simulink model "sensorExpoler"  (R2026a)
settings: Solver=FixedStepDiscrete  StopTime=inf  FixedStep=0.001
undefined symbols (not defined in the file): Blocking, Non
libraries: amg_usbconverter_n_connect_lib x2
settings Model: Creator=pboon  LastModifiedBy=Next

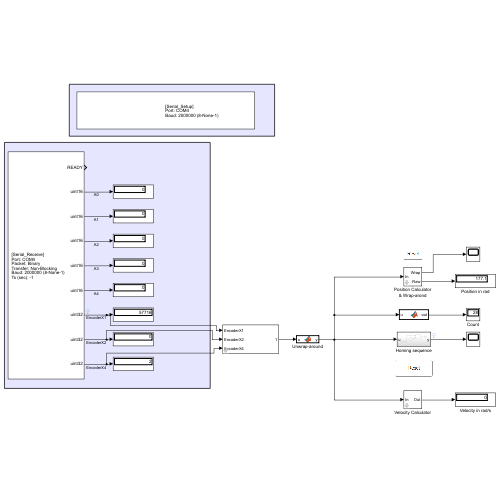
[thumbnail: Simulink's stored preview of the top-level diagram]
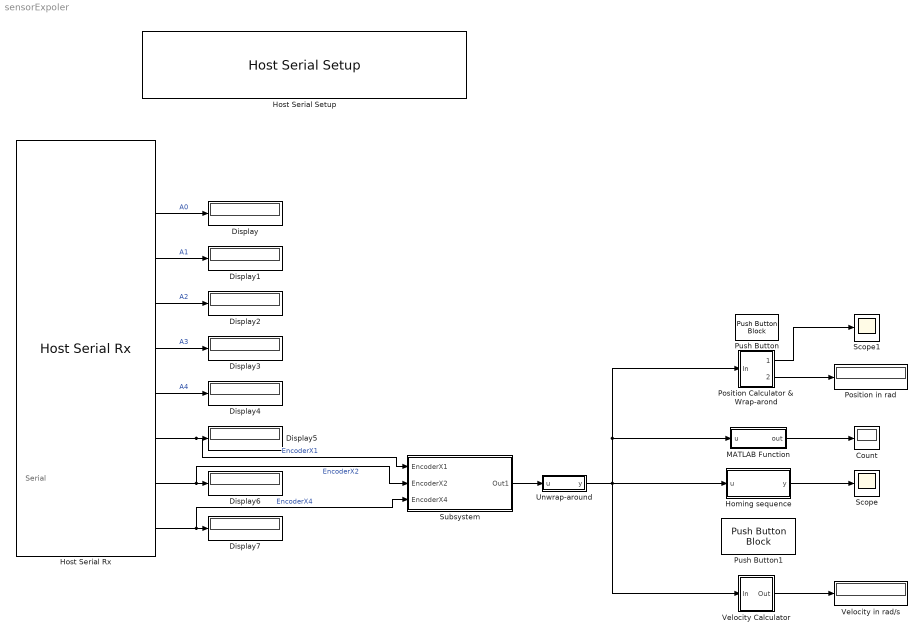
== system sensorExpoler ==
  note: Serial
  Count : Display
  Display{,1..7} (8 alike) : Display
      Display5 settings: Format=decimal (Stored Integer)
      Display6 settings: Format=decimal (Stored Integer)
      Display7 settings: Format=decimal (Stored Integer)
  Homing sequence : Subsystem
  Host Serial Rx : amg_usbconverter_n_connect_lib/Host Serial Rx  conf=rx  port=COM4  baudrate=2000000  databits=8  parity=None  stopbit=1  flowcontrol=None  transfer=Non-Blocking  timeout=5  packetmode=Binary  enableinitialvalues=off  initialvalues=[]  binheader='25'  binterminator='4E 4E'  porttype_double=0  porttype_single=0  porttype_int8=0  porttype_uint8=0  porttype_int16=0  porttype_uint16=5  porttype_int32=0  porttype_uint32=3  asciiformat='%d,%f'  rx_asciiterminator="CRLF (0x0D 0x0A - \"\\r\\n\")"  tx_asciiterminator="CRLF (0x0D 0x0A - \"\\r\\n\")"  sampletime=0.001  enablecustomportlabel=off  cinputportlabel=0  coutputportlabel=A  portpinstr=0  blockid=HostSerialRx  inputporttype=[]  inputportwidth=[]  inputportlabel={}  outputporttype=[3 5 5 5 5 5 7 7 7]  outputportwidth=[1 1 1 1 1 1 1 1 1]  outputportlabel={'READY','uint16','uint16','uint16','uint16','uint16','uint32','uint32','uint32'}  compat=0  optionstring=[]  autoport='COM4'
  Host Serial Setup : amg_usbconverter_n_connect_lib/Host Serial Setup  conf=setup  port=COM4  baudrate=2000000  databits=8  parity=None  stopbit=1  flowcontrol=None  transfer=Blocking  timeout=2  packetmode=Binary  initialvalues=[]  binheader='7E 7E'  binterminator='03 03'  porttype_double=0  porttype_single=1  porttype_int8=0  porttype_uint8=0  porttype_int16=0  porttype_uint16=0  porttype_int32=0  porttype_uint32=2  asciiformat='%d %u %x'  rx_asciiterminator="CRLF (0x0D 0x0A - \"\\r\\n\")"  tx_asciiterminator="CRLF (0x0D 0x0A - \"\\r\\n\")"  sampletime=-1  enablecustomportlabel=off  cinputportlabel=0  coutputportlabel=A  portpinstr=0  blockid=HostSerialSetup  inputporttype=[]  inputportwidth=[]  inputportlabel={}  outputporttype=[]  outputportwidth=[]  outputportlabel={}  compat=0  optionstring=[]  autoport='COM4'
  MATLAB Function : MATLAB Function  TreatAsAtomicUnit=on
  Position Calculator & Wrap-arond : Subsystem  mask{PPR=EncoderX2}
      mask prompts: PPR "Pulse per revolution"
  Position in rad : Display
  Push Button : PushButtonBlock  ButtonText=Reset  IconOnColor=[0.0, 0.39215686274509803, 0.0]  IconOffColor=[0.0, 1.0, 0.0]  OffValue=0.000000
  Push Button1 : PushButtonBlock  ButtonText=Reset  IconOnColor=[0.0, 0.39215686274509803, 0.0]  IconOffColor=[0.0, 1.0, 0.0]  OffValue=0.000000
  Scope : Scope
      settings: ActiveDisplayYMinimum=-505040.01657105918  ActiveDisplayYMaximum=287658.22323698009
  Scope1 : Scope
      settings: ActiveDisplayYMinimum=-4.6888606130862911  ActiveDisplayYMaximum=11.610473252660341
  Subsystem : Subsystem  mask{set=EncoderX2}
      mask prompts: set "Select encoding mode"
  Unwrap-around : MATLAB Function  TreatAsAtomicUnit=on
  Velocity Calculator : Subsystem  mask{PPR=EncoderX2}
      mask prompts: PPR "Pulse per revolution for"
  Velocity in rad/s : Display
  wires:
  Host Serial Rx/2 -> Display/1  "A0"
  Host Serial Rx/3 -> Display1/1  "A1"
  Host Serial Rx/4 -> Display2/1  "A2"
  Host Serial Rx/5 -> Display3/1  "A3"
  Host Serial Rx/6 -> Display4/1  "A4"
  Host Serial Rx/7 -> Subsystem/1(EncoderX1), Display5/1  "EncoderX1"
  Host Serial Rx/8 -> Subsystem/2(EncoderX2), Display6/1  "EncoderX2"
  Host Serial Rx/9 -> Subsystem/3(EncoderX4), Display7/1  "EncoderX4"
  Position Calculator & Wrap-arond/1(Wrap) -> Scope1/1
  Position Calculator & Wrap-arond/2(Raw) -> Position in rad/1
  Velocity Calculator/1(Out) -> Velocity in rad/s/1
  Subsystem/1(Out1) -> Unwrap-around/1(u)
  Homing sequence/1(y) -> Scope/1
  MATLAB Function/1(out) -> Count/1
  Unwrap-around/1(y) -> MATLAB Function/1(u), Position Calculator & Wrap-arond/1(In), Homing sequence/1(u), Velocity Calculator/1(In)

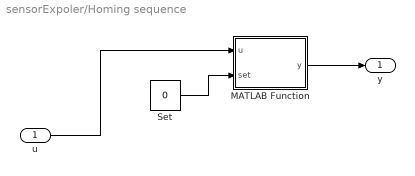
== system sensorExpoler/Homing sequence ==
  u : Inport
  MATLAB Function : MATLAB Function  TreatAsAtomicUnit=on
  Set : Constant  Value=0
  y : Outport
  wires:
  u/1 -> MATLAB Function/1(u)
  Set/1 -> MATLAB Function/2(set)
  MATLAB Function/1(y) -> y/1

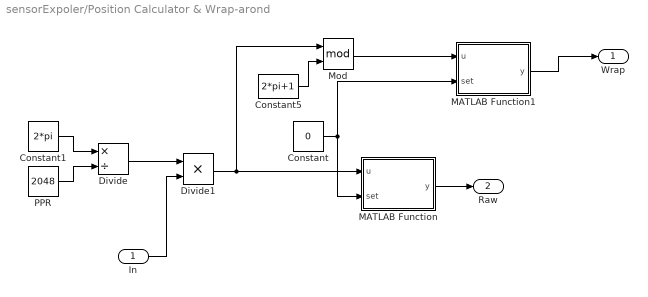
== system sensorExpoler/Position Calculator & Wrap-arond ==
  In : Inport
  Constant : Constant  Value=0
  Constant1 : Constant  Value=2*pi
  Constant5 : Constant  Value=2*pi+1
  Divide : Product  Inputs=*/
  Divide1 : Product  Inputs=**
  MATLAB Function : MATLAB Function  TreatAsAtomicUnit=on
  MATLAB Function1 : MATLAB Function  TreatAsAtomicUnit=on
  Mod : Math  Operator=mod
  PPR : Constant  Value=2048
  Wrap : Outport
  Raw : Outport  Port=2
  wires:
  Constant1/1 -> Divide/1
  Divide1/1 -> MATLAB Function/1(u), Mod/1
  Divide/1 -> Divide1/1
  PPR/1 -> Divide/2
  Constant5/1 -> Mod/2
  In/1 -> Divide1/2
  Constant/1 -> MATLAB Function1/2(set), MATLAB Function/2(set)
  MATLAB Function/1(y) -> Raw/1
  Mod/1 -> MATLAB Function1/1(u)
  MATLAB Function1/1(y) -> Wrap/1

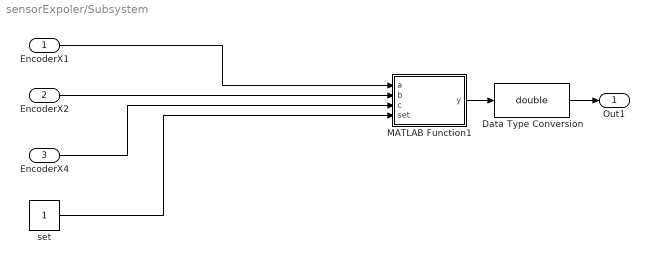
== system sensorExpoler/Subsystem ==
  EncoderX1 : Inport
  EncoderX2 : Inport  Port=2
  EncoderX4 : Inport  Port=3
  Data Type Conversion : DataTypeConversion  OutDataTypeStr=double  SaturateOnIntegerOverflow=off  RndMeth=Floor
  MATLAB Function1 : MATLAB Function  TreatAsAtomicUnit=on
  set : Constant
  Out1 : Outport
  wires:
  MATLAB Function1/1(y) -> Data Type Conversion/1
  EncoderX2/1 -> MATLAB Function1/2(b)
  EncoderX1/1 -> MATLAB Function1/1(a)
  Data Type Conversion/1 -> Out1/1
  EncoderX4/1 -> MATLAB Function1/3(c)
  set/1 -> MATLAB Function1/4(set)

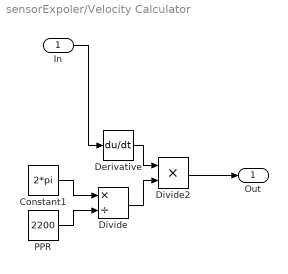
== system sensorExpoler/Velocity Calculator ==
  In : Inport
  Constant1 : Constant  Value=2*pi
  Derivative : Derivative
  Divide : Product  Inputs=*/
  Divide2 : Product  Inputs=**
  PPR : Constant  Value=2200
  Out : Outport
  wires:
  Divide2/1 -> Out/1
  Derivative/1 -> Divide2/1
  Constant1/1 -> Divide/1
  PPR/1 -> Divide/2
  Divide/1 -> Divide2/2
  In/1 -> Derivative/1

== matlab function sensorExpoler/Subsystem/MATLAB Function1 ==
  data: a input; y output; b input; c input; set input
function y = fcn(a,b,c, set)

if(set == 1)
       y = a;
elseif (set == 2)
       y = b;
else
    y = c;

end

== matlab function sensorExpoler/Homing sequence/MATLAB Function ==
  data: u input; y output; set input
function y = fcn(u, set)

persistent tareValue

if isempty(tareValue)
    tareValue = 0;
end

% Tare
if set == 1
    tareValue = u-1;
end

% Wrap-around after subtracting tare
y = mod(u - tareValue,u + 1);

== matlab function sensorExpoler/Position Calculator & Wrap-arond/MATLAB Function ==
  data: u input; y output; set input
function y = fcn(u, set)

persistent tare

if isempty(tare)
    tare = 0;
end

if set
    tare = u;
end

y = u - tare;

== matlab function sensorExpoler/Position Calculator & Wrap-arond/MATLAB Function1 ==
  data: u input; y output; set input
function y = fcn(u, set)

persistent tare

if isempty(tare)
    tare = 0;
end

if set
    tare = u;
end

y = u - tare;

== matlab function sensorExpoler/MATLAB Function ==
  data: u input; out output
function out= fcn(u)

out = floor(u/2048);
% 2048
% 4096
% 8192

== matlab function sensorExpoler/Unwrap-around ==
  data: u input; y output
function y = fcn(u)

persistent prev y0

if isempty(prev)
    prev = u;
    y0 = u;
end

delta = u - prev;

if delta > 32768
    delta = delta - 65536;
elseif delta < -32768
    delta = delta + 65536;
end

y0 = y0 + delta;
y = y0;

prev = u;
